simulink library "IEEE_39Bus_dynload_lib"  (Simulink 8.5)
settings: Solver=ode45  StartTime=0.0  StopTime=10.0  RelTol=1e-3
libraries: powerlib_meascontrol x1, dspstat3 x1
settings Model: Creator=Administrator  LastModifiedBy=Administrator

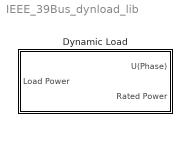
== system IEEE_39Bus_dynload_lib ==
  Dynamic Load : Subsystem  mask(Daynamic Load from EPRI LOADSYN){Kpf=1, Kpv=1.7, Kqf=-1.7, Kqv=2.6, Fnom=50, winlen=240}
      mask prompts: Fnom "Nominal Frequency [Hz]"; winlen "Window Length (ms)"
      mask help:
      | P=P0*(V/V0)*[Kpv * [1+Kpf(f-f0)]
      | Q=Q0*(V/V0)*[Kqv*(1+Kqf(f-f0)]
      |
      | PLL measured frequency and RMS voltage value are filtered

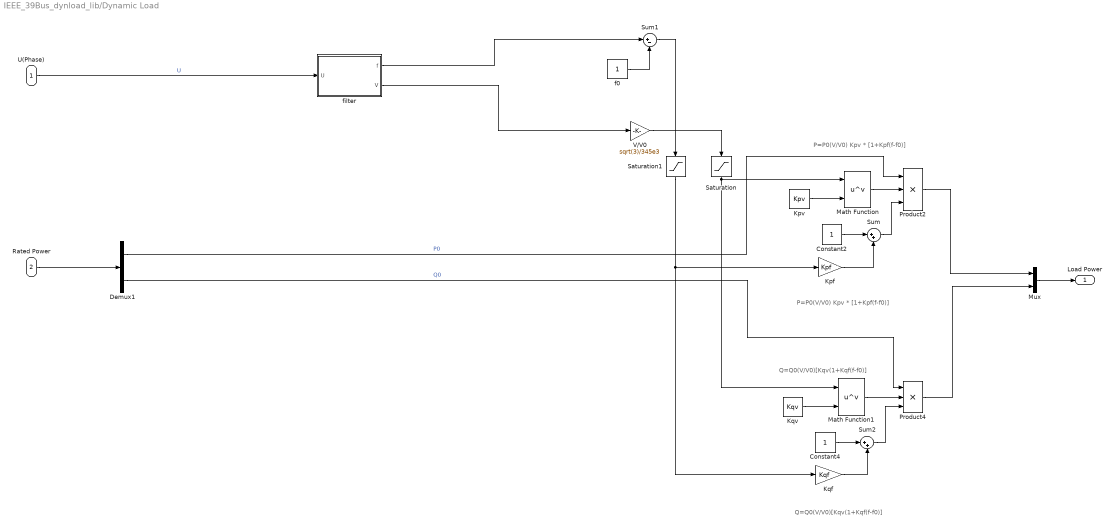
== system IEEE_39Bus_dynload_lib/Dynamic Load ==
  note: P=P0(V/V0) Kpv * [1+Kpf(f-f0)]
  note: Q=Q0(V/V0)[Kqv(1+Kqf(f-f0)]
  note: Q=Q0(V/V0)[Kqv(1+Kqf(f-f0)]
  note: P=P0(V/V0) Kpv * [1+Kpf(f-f0)]
  U(Phase) : Inport
  Rated Power : Inport  Port=2
  Constant2 : Constant
  Constant4 : Constant
  Demux1 : Demux  Outputs=2
  Kpf : Gain  Gain=Kpf
  Kpv : Constant  Value=Kpv
  Kqf : Gain  Gain=Kqf
  Kqv : Constant  Value=Kqv
  Math Function : Math  Operator=pow  SaturateOnIntegerOverflow=on
  Math Function1 : Math  Operator=pow  SaturateOnIntegerOverflow=on
  Mux : Mux  Inputs=2
  Product2 : Product  Inputs=3
  Product4 : Product  Inputs=3
  Saturation : Saturate  UpperLimit=1.5  LowerLimit=0
  Saturation1 : Saturate  UpperLimit=2  LowerLimit=-3
  Sum : Sum  Inputs=|++
  Sum1 : Sum  Inputs=|+-
  Sum2 : Sum  Inputs=|++
  V/V0 : Gain  Gain=sqrt(3)/345e3
  f0 : Constant
  "filter " : Subsystem
  Load Power : Outport
  wires:
  Product2/1 -> Mux/1
  Demux1/1 -> Product2/1  "P0"
  V/V0/1 -> Saturation/1
  Kpv/1 -> Math Function/2
  Math Function/1 -> Product2/2
  Sum/1 -> Product2/3
  Constant2/1 -> Sum/1
  f0/1 -> Sum1/2
  Kpf/1 -> Sum/2
  Demux1/2 -> Product4/1  "Q0"
  Kqv/1 -> Math Function1/2
  Math Function1/1 -> Product4/2
  Sum2/1 -> Product4/3
  Constant4/1 -> Sum2/1
  Kqf/1 -> Sum2/2
  Product4/1 -> Mux/2
  Saturation/1 -> Math Function/1, Math Function1/1
  Saturation1/1 -> Kpf/1, Kqf/1
  Rated Power/1 -> Demux1/1
  Sum1/1 -> Saturation1/1
  Mux/1 -> Load Power/1
  U(Phase)/1 -> "filter "/1(U)  "U"
  "filter "/1(f) -> Sum1/1
  "filter "/2(V) -> V/V0/1

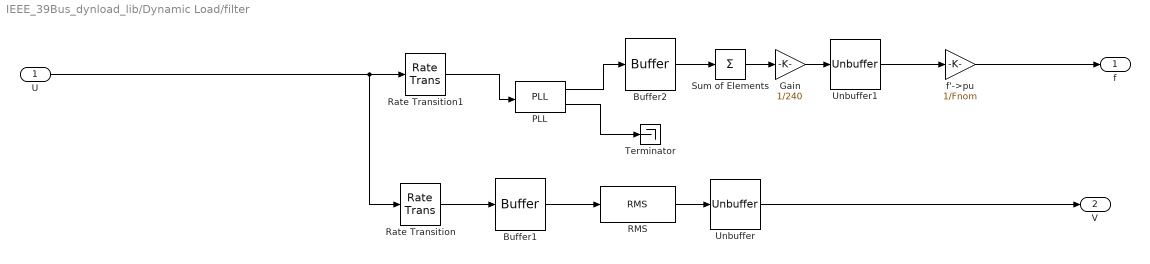
== system IEEE_39Bus_dynload_lib/Dynamic Load/filter  ==
  U : Inport
  Buffer1 : Buffer  N=winlen*10  V=(winlen-20)*10  TreatMby1Signals=One channel
  Buffer2 : Buffer  N=winlen  V=winlen-20  TreatMby1Signals=One channel
  Gain : Gain  Gain=1/240
  PLL : powerlib_meascontrol/PLL/PLL  Fmin=45  Par_Init=[0, 50]  ParK=[180, 3200, 1]  TcD=1e-3  MaxRateChangeFreq=25  FilterCutOffFreq=25  Ts=1e-3  AGC=on
  RMS : dspstat3/RMS  run=off  reset_popup=None  InputProcessing=Columns as channels (frame based)  directionMode=Each column  dimension=1  treatSBRowAsCol=off
  Rate Transition : RateTransition  Integrity=off  Deterministic=off  OutPortSampleTime=100e-6
  Rate Transition1 : RateTransition  Integrity=off  Deterministic=off  OutPortSampleTime=100e-6
  Sum of Elements : Sum  Inputs=+
  Terminator : Terminator
  Unbuffer : Unbuffer  SampleBasedProcessing=Same as frame based
  Unbuffer1 : Unbuffer  SampleBasedProcessing=Same as frame based
  f'->pu : Gain  Gain=1/Fnom
  f : Outport
  V : Outport  Port=2
  wires:
  Unbuffer1/1 -> f'->pu/1
  f'->pu/1 -> f/1
  Unbuffer/1 -> V/1
  Rate Transition1/1 -> PLL/1
  Rate Transition/1 -> Buffer1/1
  Gain/1 -> Unbuffer1/1
  Sum of Elements/1 -> Gain/1
  Buffer2/1 -> Sum of Elements/1
  PLL/1 -> Buffer2/1
  U/1 -> Rate Transition/1, Rate Transition1/1
  PLL/2 -> Terminator/1
  RMS/1 -> Unbuffer/1
  Buffer1/1 -> RMS/1
